simulink subsystem "Traffic_info29"  (R2022b)
settings: Solver=VariableStepAuto  StartTime=0.0  StopTime=10.0  RelTol=1e-3
libraries: CarMaker4SL x29
settings Model: Creator=user  LastModifiedBy=user

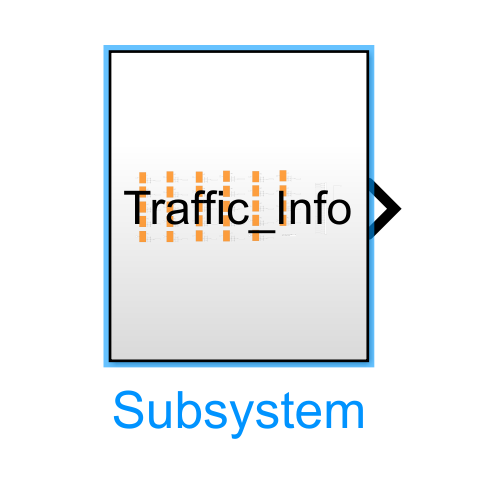
[thumbnail: Simulink's stored preview of the top-level diagram]
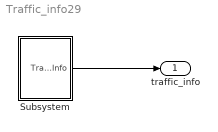
== system Traffic_info29 ==
  Subsystem : Subsystem
  traffic_info : Outport
  wires:
  Subsystem/1(Traffic_Info) -> traffic_info/1

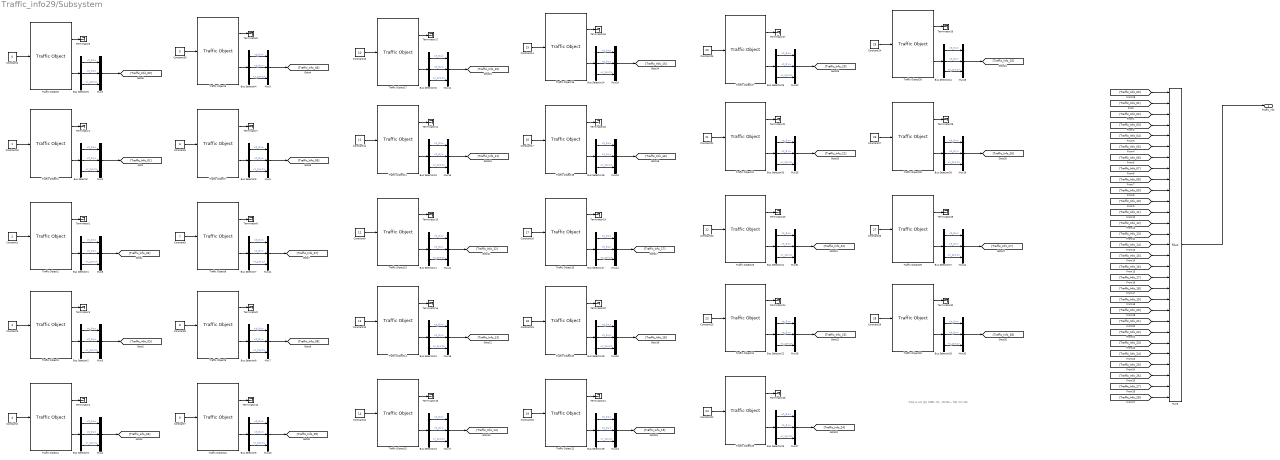
== system Traffic_info29/Subsystem ==
  note: 주차장 & 도로 합친 traffic 개수 : 29
      | T00 ~ T28까지 Info
  Bus Selector{,1..28} (29 alike) : BusSelector  OutputSignals=t_0 x,t_0 y,r_zyx z
  Constant1 : Constant  Value=2
  Constant10 : Constant
  Constant11 : Constant  Value=11
  Constant12 : Constant  Value=14
  Constant13 : Constant  Value=13
  Constant14 : Constant  Value=15
  Constant15 : Constant  Value=10
  Constant16 : Constant  Value=17
  Constant17 : Constant  Value=16
  Constant18 : Constant  Value=19
  Constant19 : Constant  Value=18
  Constant2 : Constant  Value=4
  Constant20 : Constant  Value=22
  Constant21 : Constant  Value=21
  Constant22 : Constant  Value=24
  Constant23 : Constant  Value=23
  Constant24 : Constant  Value=25
  Constant25 : Constant  Value=20
  Constant26 : Constant  Value=27
  Constant27 : Constant  Value=26
  Constant29 : Constant  Value=28
  Constant3 : Constant  Value=3
  Constant30 : Constant  Value=5
  Constant4 : Constant  Value=0
  Constant5 : Constant  Value=7
  Constant6 : Constant  Value=6
  Constant7 : Constant  Value=9
  Constant8 : Constant  Value=8
  Constant9 : Constant  Value=12
  Mux{1..8,10..22,24..31} (29 alike) : Mux  Inputs=3
  Mux9 : Mux  Inputs=29
  Terminator{1..21,23..30} (29 alike) : Terminator
  Traffic Object1 : CarMaker4SL/Traffic Object  xname=T01  ximode=Traffic Id  xstime=Inherited
      settings: SourceProductName=CarMaker4SL
  Traffic Object10 : CarMaker4SL/Traffic Object  xname=T09  ximode=Traffic Id  xstime=Inherited
      settings: SourceProductName=CarMaker4SL
  Traffic Object11 : CarMaker4SL/Traffic Object  xname=T11  ximode=Traffic Id  xstime=Inherited
      settings: SourceProductName=CarMaker4SL
  Traffic Object12 : CarMaker4SL/Traffic Object  xname=T19  ximode=Traffic Id  xstime=Inherited
      settings: SourceProductName=CarMaker4SL
  Traffic Object13 : CarMaker4SL/Traffic Object  xname=T12  ximode=Traffic Id  xstime=Inherited
      settings: SourceProductName=CarMaker4SL
  Traffic Object14 : CarMaker4SL/Traffic Object  xname=T13  ximode=Traffic Id  xstime=Inherited
      settings: SourceProductName=CarMaker4SL
  Traffic Object15 : CarMaker4SL/Traffic Object  xname=T14  ximode=Traffic Id  xstime=Inherited
      settings: SourceProductName=CarMaker4SL
  Traffic Object16 : CarMaker4SL/Traffic Object  xname=T15  ximode=Traffic Id  xstime=Inherited
      settings: SourceProductName=CarMaker4SL
  Traffic Object17 : CarMaker4SL/Traffic Object  xname=T10  ximode=Traffic Id  xstime=Inherited
      settings: SourceProductName=CarMaker4SL
  Traffic Object18 : CarMaker4SL/Traffic Object  xname=T16  ximode=Traffic Id  xstime=Inherited
      settings: SourceProductName=CarMaker4SL
  Traffic Object19 : CarMaker4SL/Traffic Object  xname=T17  ximode=Traffic Id  xstime=Inherited
      settings: SourceProductName=CarMaker4SL
  Traffic Object2 : CarMaker4SL/Traffic Object  xname=T02  ximode=Traffic Id  xstime=Inherited
      settings: SourceProductName=CarMaker4SL
  Traffic Object20 : CarMaker4SL/Traffic Object  xname=T18  ximode=Traffic Id  xstime=Inherited
      settings: SourceProductName=CarMaker4SL
  Traffic Object21 : CarMaker4SL/Traffic Object  xname=T21  ximode=Traffic Id  xstime=Inherited
      settings: SourceProductName=CarMaker4SL
  Traffic Object23 : CarMaker4SL/Traffic Object  xname=T22  ximode=Traffic Id  xstime=Inherited
      settings: SourceProductName=CarMaker4SL
  Traffic Object24 : CarMaker4SL/Traffic Object  xname=T23  ximode=Traffic Id  xstime=Inherited
      settings: SourceProductName=CarMaker4SL
  Traffic Object25 : CarMaker4SL/Traffic Object  xname=T24  ximode=Traffic Id  xstime=Inherited
      settings: SourceProductName=CarMaker4SL
  Traffic Object26 : CarMaker4SL/Traffic Object  xname=T25  ximode=Traffic Id  xstime=Inherited
      settings: SourceProductName=CarMaker4SL
  Traffic Object27 : CarMaker4SL/Traffic Object  xname=T20  ximode=Traffic Id  xstime=Inherited
      settings: SourceProductName=CarMaker4SL
  Traffic Object28 : CarMaker4SL/Traffic Object  xname=T26  ximode=Traffic Id  xstime=Inherited
      settings: SourceProductName=CarMaker4SL
  Traffic Object29 : CarMaker4SL/Traffic Object  xname=T27  ximode=Traffic Id  xstime=Inherited
      settings: SourceProductName=CarMaker4SL
  Traffic Object3 : CarMaker4SL/Traffic Object  xname=T03  ximode=Traffic Id  xstime=Inherited
      settings: SourceProductName=CarMaker4SL
  Traffic Object30 : CarMaker4SL/Traffic Object  xname=T28  ximode=Traffic Id  xstime=Inherited
      settings: SourceProductName=CarMaker4SL
  Traffic Object4 : CarMaker4SL/Traffic Object  xname=T04  ximode=Traffic Id  xstime=Inherited
      settings: SourceProductName=CarMaker4SL
  Traffic Object5 : CarMaker4SL/Traffic Object  xname=T05  ximode=Traffic Id  xstime=Inherited
      settings: SourceProductName=CarMaker4SL
  Traffic Object6 : CarMaker4SL/Traffic Object  xname=T00  ximode=Traffic Id  xstime=Inherited
      settings: SourceProductName=CarMaker4SL
  Traffic Object7 : CarMaker4SL/Traffic Object  xname=T06  ximode=Traffic Id  xstime=Inherited
      settings: SourceProductName=CarMaker4SL
  Traffic Object8 : CarMaker4SL/Traffic Object  xname=T07  ximode=Traffic Id  xstime=Inherited
      settings: SourceProductName=CarMaker4SL
  Traffic Object9 : CarMaker4SL/Traffic Object  xname=T08  ximode=Traffic Id  xstime=Inherited
      settings: SourceProductName=CarMaker4SL
  Traffic_Info : Outport
  wires:
  Bus Selector15/2 -> Mux12/2  "<t_0 y>"
  Bus Selector15/3 -> Mux12/3  "<r_zyx z>"
  Traffic Object9/1 -> Terminator9/1
  Traffic Object21/2 -> Bus Selector20/1
  Bus Selector4/3 -> Mux5/3  "<r_zyx z>"
  Constant12/1 -> Traffic Object15/1
  Mux27/1 -> [Traffic_Info_24]
  Traffic Object1/1 -> Terminator1/1
  Traffic Object4/2 -> Bus Selector3/1
  Bus Selector3/2 -> Mux4/2  "<t_0 y>"
  Bus Selector14/3 -> Mux18/3  "<r_zyx z>"
  [Traffic_Info_24] -> Mux9/25
  Bus Selector16/2 -> Mux19/2  "<t_0 y>"
  Mux17/1 -> [Traffic_Info_14]
  Bus Selector13/1 -> Mux17/1  "<t_0 x>"
  Mux8/1 -> [Traffic_Info_02]
  Bus Selector18/2 -> Mux20/2  "<t_0 y>"
  Mux15/1 -> [Traffic_Info_11]
  Traffic Object2/2 -> Bus Selector1/1
  Bus Selector12/3 -> Mux16/3  "<r_zyx z>"
  [Traffic_Info_25] -> Mux9/26
  Mux16/1 -> [Traffic_Info_13]
  Mux9/1 -> Traffic_Info/1
  Bus Selector23/1 -> Mux27/1  "<t_0 x>"
  Bus Selector1/3 -> Mux8/3  "<r_zyx z>"
  Bus Selector25/2 -> Mux22/2  "<t_0 y>"
  Bus Selector20/3 -> Mux25/3  "<r_zyx z>"
  Mux2/1 -> [Traffic_Info_01]
  [Traffic_Info_18] -> Mux9/19
  Bus Selector18/3 -> Mux20/3  "<r_zyx z>"
  [Traffic_Info_19] -> Mux9/20
  Traffic Object16/2 -> Bus Selector14/1
  Bus Selector10/3 -> Mux15/3  "<r_zyx z>"
  Bus Selector15/1 -> Mux12/1  "<t_0 x>"
  [Traffic_Info_20] -> Mux9/21
  Traffic Object14/2 -> Bus Selector12/1
  Constant27/1 -> Traffic Object28/1
  Traffic Object7/1 -> Terminator7/1
  Constant20/1 -> Traffic Object23/1
  Bus Selector/2 -> Mux2/2  "<t_0 y>"
  Mux26/1 -> [Traffic_Info_23]
  Mux4/1 -> [Traffic_Info_04]
  Bus Selector27/2 -> Mux24/2  "<t_0 y>"
  [Traffic_Info_17] -> Mux9/18
  Bus Selector24/2 -> Mux28/2  "<t_0 y>"
  [Traffic_Info_15] -> Mux9/16
  [Traffic_Info_09] -> Mux9/10
  Bus Selector2/1 -> Mux3/1  "<t_0 x>"
  Constant10/1 -> Traffic Object1/1
  Traffic Object23/1 -> Terminator23/1
  [Traffic_Info_14] -> Mux9/15
  Constant3/1 -> Traffic Object3/1
  Traffic Object4/1 -> Terminator4/1
  Constant14/1 -> Traffic Object16/1
  Traffic Object18/2 -> Bus Selector16/1
  Traffic Object14/1 -> Terminator14/1
  Mux18/1 -> [Traffic_Info_15]
  Bus Selector14/2 -> Mux18/2  "<t_0 y>"
  [Traffic_Info_05] -> Mux9/6
  Constant2/1 -> Traffic Object4/1
  Mux11/1 -> [Traffic_Info_07]
  Traffic Object19/1 -> Terminator19/1
  Traffic Object15/1 -> Terminator15/1
  Bus Selector20/1 -> Mux25/1  "<t_0 x>"
  Bus Selector27/1 -> Mux24/1  "<t_0 x>"
  [Traffic_Info_07] -> Mux9/8
  Constant15/1 -> Traffic Object17/1
  Traffic Object5/2 -> Bus Selector4/1
  Mux31/1 -> [Traffic_Info_22]
  Traffic Object1/2 -> Bus Selector/1
  [Traffic_Info_22] -> Mux9/23
  Bus Selector8/2 -> Mux7/2  "<t_0 y>"
  Bus Selector1/1 -> Mux8/1  "<t_0 x>"
  Traffic Object3/1 -> Terminator3/1
  Mux12/1 -> [Traffic_Info_10]
  Traffic Object17/2 -> Bus Selector15/1
  Bus Selector14/1 -> Mux18/1  "<t_0 x>"
  Bus Selector24/1 -> Mux28/1  "<t_0 x>"
  Bus Selector2/2 -> Mux3/2  "<t_0 y>"
  Bus Selector2/3 -> Mux3/3  "<r_zyx z>"
  Bus Selector8/1 -> Mux7/1  "<t_0 x>"
  Traffic Object2/1 -> Terminator2/1
  Constant1/1 -> Traffic Object2/1
  Bus Selector/1 -> Mux2/1  "<t_0 x>"
  Bus Selector1/2 -> Mux8/2  "<t_0 y>"
  Bus Selector/3 -> Mux2/3  "<r_zyx z>"
  Mux22/1 -> [Traffic_Info_20]
  Bus Selector25/1 -> Mux22/1  "<t_0 x>"
  Bus Selector13/2 -> Mux17/2  "<t_0 y>"
  Constant9/1 -> Traffic Object13/1
  Bus Selector17/2 -> Mux14/2  "<t_0 y>"
  Bus Selector19/2 -> Mux13/2  "<t_0 y>"
  Traffic Object13/2 -> Bus Selector11/1
  Constant29/1 -> Traffic Object30/1
  Traffic Object3/2 -> Bus Selector2/1
  Bus Selector8/3 -> Mux7/3  "<r_zyx z>"
  Bus Selector16/3 -> Mux19/3  "<r_zyx z>"
  Constant13/1 -> Traffic Object14/1
  Bus Selector23/3 -> Mux27/3  "<r_zyx z>"
  Traffic Object12/2 -> Bus Selector19/1
  Bus Selector12/2 -> Mux16/2  "<t_0 y>"
  Traffic Object13/1 -> Terminator13/1
  Bus Selector7/3 -> Mux11/3  "<r_zyx z>"
  Bus Selector18/1 -> Mux20/1  "<t_0 x>"
  Bus Selector7/2 -> Mux11/2  "<t_0 y>"
  Traffic Object5/1 -> Terminator5/1
  Traffic Object20/2 -> Bus Selector18/1
  Mux14/1 -> [Traffic_Info_17]
  Bus Selector11/3 -> Mux21/3  "<r_zyx z>"
  Mux21/1 -> [Traffic_Info_12]
  Bus Selector16/1 -> Mux19/1  "<t_0 x>"
  Traffic Object20/1 -> Terminator20/1
  Traffic Object15/2 -> Bus Selector13/1
  Constant16/1 -> Traffic Object19/1
  Mux20/1 -> [Traffic_Info_18]
  Traffic Object12/1 -> Terminator12/1
  Traffic Object11/1 -> Terminator11/1
  Bus Selector10/2 -> Mux15/2  "<t_0 y>"
  Bus Selector11/2 -> Mux21/2  "<t_0 y>"
  Bus Selector10/1 -> Mux15/1  "<t_0 x>"
  Bus Selector11/1 -> Mux21/1  "<t_0 x>"
  Traffic Object11/2 -> Bus Selector10/1
  Traffic Object17/1 -> Terminator17/1
  Constant8/1 -> Traffic Object9/1
  Constant6/1 -> Traffic Object7/1
  Constant7/1 -> Traffic Object10/1
  Traffic Object10/1 -> Terminator10/1
  [Traffic_Info_08] -> Mux9/9
  Mux6/1 -> [Traffic_Info_06]
  Bus Selector4/1 -> Mux5/1  "<t_0 x>"
  Traffic Object10/2 -> Bus Selector9/1
  Bus Selector20/2 -> Mux25/2  "<t_0 y>"
  [Traffic_Info_27] -> Mux9/28
  Bus Selector9/3 -> Mux10/3  "<r_zyx z>"
  Mux10/1 -> [Traffic_Info_09]
  Bus Selector9/1 -> Mux10/1  "<t_0 x>"
  Mux7/1 -> [Traffic_Info_08]
  Traffic Object9/2 -> Bus Selector8/1
  Bus Selector6/3 -> Mux6/3  "<r_zyx z>"
  Bus Selector13/3 -> Mux17/3  "<r_zyx z>"
  Bus Selector6/2 -> Mux6/2  "<t_0 y>"
  [Traffic_Info_10] -> Mux9/11
  Bus Selector4/2 -> Mux5/2  "<t_0 y>"
  Constant5/1 -> Traffic Object8/1
  Traffic Object8/1 -> Terminator8/1
  Bus Selector9/2 -> Mux10/2  "<t_0 y>"
  Bus Selector28/1 -> Mux30/1  "<t_0 x>"
  Traffic Object7/2 -> Bus Selector6/1
  Bus Selector6/1 -> Mux6/1  "<t_0 x>"
  Traffic Object6/2 -> Bus Selector5/1
  Bus Selector7/1 -> Mux11/1  "<t_0 x>"
  [Traffic_Info_06] -> Mux9/7
  Traffic Object8/2 -> Bus Selector7/1
  Traffic Object16/1 -> Terminator16/1
  [Traffic_Info_11] -> Mux9/12
  Traffic Object27/2 -> Bus Selector25/1
  [Traffic_Info_03] -> Mux9/4
  [Traffic_Info_28] -> Mux9/29
  [Traffic_Info_02] -> Mux9/3
  Mux3/1 -> [Traffic_Info_03]
  Bus Selector3/1 -> Mux4/1  "<t_0 x>"
  Bus Selector3/3 -> Mux4/3  "<r_zyx z>"
  Traffic Object19/2 -> Bus Selector17/1
  Bus Selector17/1 -> Mux14/1  "<t_0 x>"
  Constant11/1 -> Traffic Object11/1
  Bus Selector5/3 -> Mux1/3  "<r_zyx z>"
  Constant19/1 -> Traffic Object20/1
  Traffic Object26/1 -> Terminator26/1
  Constant17/1 -> Traffic Object18/1
  [Traffic_Info_04] -> Mux9/5
  Bus Selector19/1 -> Mux13/1  "<t_0 x>"
  Traffic Object18/1 -> Terminator18/1
  Mux13/1 -> [Traffic_Info_19]
  Bus Selector17/3 -> Mux14/3  "<r_zyx z>"
  [Traffic_Info_23] -> Mux9/24
  Bus Selector19/3 -> Mux13/3  "<r_zyx z>"
  Mux19/1 -> [Traffic_Info_16]
  Constant18/1 -> Traffic Object12/1
  Bus Selector23/2 -> Mux27/2  "<t_0 y>"
  Bus Selector12/1 -> Mux16/1  "<t_0 x>"
  [Traffic_Info_00] -> Mux9/1
  [Traffic_Info_16] -> Mux9/17
  Traffic Object29/2 -> Bus Selector27/1
  Constant30/1 -> Traffic Object5/1
  Bus Selector28/3 -> Mux30/3  "<r_zyx z>"
  Mux5/1 -> [Traffic_Info_05]
  [Traffic_Info_21] -> Mux9/22
  Traffic Object26/2 -> Bus Selector24/1
  Constant22/1 -> Traffic Object25/1
  Mux24/1 -> [Traffic_Info_27]
  Bus Selector22/2 -> Mux26/2  "<t_0 y>"
  Constant23/1 -> Traffic Object24/1
  Traffic Object29/1 -> Terminator29/1
  Traffic Object30/2 -> Bus Selector28/1
  Traffic Object25/2 -> Bus Selector23/1
  Bus Selector22/1 -> Mux26/1  "<t_0 x>"
  Traffic Object23/2 -> Bus Selector21/1
  Bus Selector21/3 -> Mux31/3  "<r_zyx z>"
  Traffic Object30/1 -> Terminator30/1
  Bus Selector25/3 -> Mux22/3  "<r_zyx z>"
  Constant25/1 -> Traffic Object27/1
  Traffic Object27/1 -> Terminator27/1
  Constant24/1 -> Traffic Object26/1
  Mux28/1 -> [Traffic_Info_25]
  Bus Selector21/1 -> Mux31/1  "<t_0 x>"
  Traffic Object24/1 -> Terminator24/1
  Traffic Object25/1 -> Terminator25/1
  Bus Selector26/1 -> Mux29/1  "<t_0 x>"
  Traffic Object24/2 -> Bus Selector22/1
  Mux30/1 -> [Traffic_Info_28]
  Bus Selector28/2 -> Mux30/2  "<t_0 y>"
  Traffic Object28/2 -> Bus Selector26/1
  Mux29/1 -> [Traffic_Info_26]
  Bus Selector27/3 -> Mux24/3  "<r_zyx z>"
  Traffic Object28/1 -> Terminator28/1
  Constant21/1 -> Traffic Object21/1
  Traffic Object21/1 -> Terminator21/1
  Bus Selector26/2 -> Mux29/2  "<t_0 y>"
  Constant26/1 -> Traffic Object29/1
  Bus Selector21/2 -> Mux31/2  "<t_0 y>"
  Bus Selector22/3 -> Mux26/3  "<r_zyx z>"
  Bus Selector26/3 -> Mux29/3  "<r_zyx z>"
  Bus Selector24/3 -> Mux28/3  "<r_zyx z>"
  Mux25/1 -> [Traffic_Info_21]
  [Traffic_Info_12] -> Mux9/13
  Traffic Object6/1 -> Terminator6/1
  Constant4/1 -> Traffic Object6/1
  [Traffic_Info_01] -> Mux9/2
  Bus Selector5/2 -> Mux1/2  "<t_0 y>"
  Mux1/1 -> [Traffic_Info_00]
  Bus Selector5/1 -> Mux1/1  "<t_0 x>"
  [Traffic_Info_13] -> Mux9/14
  [Traffic_Info_26] -> Mux9/27
